simulink model "Lab6_Starter"  (R2024b)
settings: Solver=ode1  StartTime=0.0  StopTime=600  FixedStep=.002  RelTol=1e-3  EnableMultiTasking=on
InitFcn:
  | StartStop___DAC = 1
values from neighbouring files (symbols this model uses):
  Kc = 0.4    [lab6_p1_variables.mat]
  Tp = 0.0108695652174    [lab6_p1_variables.mat]
  Tz = 0.434782608696    [lab6_p1_variables.mat]
libraries: ece486lib x1
settings Model: SimulationMode=external  ExtModeTrigDuration=8  Creator=The MathWorks, Inc.  LastModifiedBy=sohumb3
settings SolverCC: AlgebraicLoopSolver=TrustRegion  MaxZcPerStep=1
settings OptimizationCC: DefaultUnderspecifiedDataType=single  EnhancedBackFolding=on  PassReuseOutputArgsAs=Individual arguments  MaxStackSize=1024  OptimizeBlockOrder=speed  DifferentSizesBufferReuse=on  OptimizationCustomize=off  EfficientTunableParamExpr=on
settings DebuggingCC: ParameterTunabilityLossMsg=error  UnconnectedInputMsg=warning  UnconnectedOutputMsg=warning  UnconnectedLineMsg=warning
settings HardwareCC: ProdBitPerChar=16  ProdBitPerInt=16  ProdBitPerPointer=32  ProdBitPerSizeT=32  ProdBitPerPtrDiffT=32  ProdLargestAtomicInteger=Integer  ProdLargestAtomicFloat=None  ProdWordSize=16  ProdLongLongMode=on  ProdHWDeviceType=Texas Instruments->C2000
settings ModelReferenceCC: EnableRefExpFcnMdlSchedulingChecks=on
settings SFSimCC: MATLABDynamicMemAlloc=off
settings RTWCC: Description=Embedded Coder  SystemTargetFile=ert.tlc  HardwareBoard=TI Delfino F28379D LaunchPad  TemplateMakefile=ert_default_tmf  GenerateReport=on  Toolchain=Texas Instruments Code Composer Studio (C2000)  GPUComputeCapability=3.5  DLArmComputeVersion=19.05
settings CodeAppCC: ForceParamTrailComments=on  IgnoreCustomStorageClasses=off  OperatorAnnotations=on  SimulinkDataObjDesc=on  SFDataObjDesc=on  InsertBlockDesc=on
settings ERTTargetCC: CodeReplacementLibrary=TI C28x  SupportContinuousTime=on  ExtModeStaticAllocSize=10000  InlinedParameterPlacement=Hierarchical  DynamicArrayContainerType=coder::array

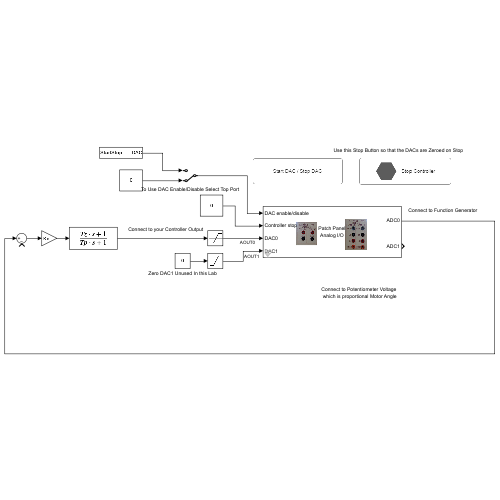
[thumbnail: Simulink's stored preview of the top-level diagram]
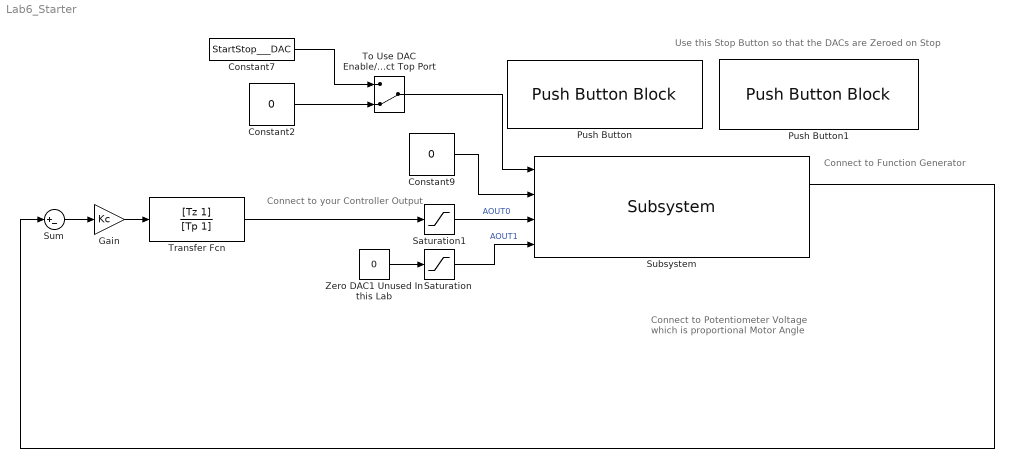
== system Lab6_Starter ==
  note: Connect to Potentiometer Voltage
      |  which is proportional Motor Angle
  note: Connect to your Controller Output
  note: Use this Stop Button so that the DACs are Zeroed on Stop
  note: Connect to Function Generator
  Constant2 : Constant  Value=0
  Constant7 : Constant  Value=StartStop___DAC
  Constant9 : Constant  Value=0
  Gain : Gain  Gain=Kc
  Push Button : PushButtonBlock  ButtonText=Start DAC / Stop DAC  OnValue=0  ButtonType=Latch  OffValue=1.000000
  Push Button1 : PushButtonBlock  ButtonText=Stop Controller  Icon=Hexagon  OffValue=0.000000
  Saturation : Saturate  UpperLimit=10  LowerLimit=-10
  Saturation1 : Saturate  UpperLimit=10  LowerLimit=-10
  Subsystem : ece486lib/Subsystem  fiexedstep=str2num(get_param(bdroot, 'FixedStep'))
  Sum : Sum  Inputs=|+-
  To Use DAC Enable/Disable Select Top Port : ManualSwitch  CurrentSetting=0
  Transfer Fcn : TransferFcn  Numerator=[Tz 1]  Denominator=[Tp 1]
  Zero DAC1 Unused In this Lab : Constant  Value=0
  wires:
  Zero DAC1 Unused In this Lab/1 -> Saturation/1
  Constant9/1 -> Subsystem/2
  Saturation1/1 -> Subsystem/3  "AOUT0"
  Saturation/1 -> Subsystem/4  "AOUT1"
  Transfer Fcn/1 -> Saturation1/1
  Constant7/1 -> To Use DAC Enable/Disable Select Top Port/1
  Constant2/1 -> To Use DAC Enable/Disable Select Top Port/2
  To Use DAC Enable/Disable Select Top Port/1 -> Subsystem/1
  Gain/1 -> Transfer Fcn/1
  Subsystem/1 -> Sum/1
  Sum/1 -> Gain/1
